simulink model "subCalc"  (R2016b)
settings: Solver=VariableStepAuto  StartTime=0.0  StopTime=10.0  RelTol=1e-3
settings Model: Creator=Radwa  LastModifiedBy=Radwa

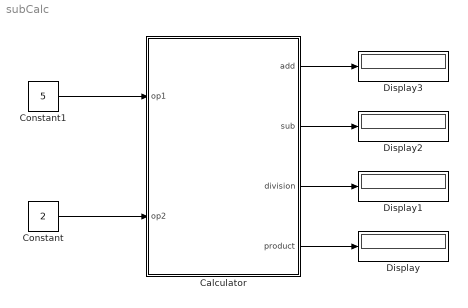
== system subCalc ==
  Calculator : Subsystem
  Constant : Constant  Value=2
  Constant1 : Constant  Value=5
  Display{,1..3} (4 alike) : Display
  wires:
  Constant1/1 -> Calculator/1(op1)
  Constant/1 -> Calculator/2(op2)
  Calculator/1(add) -> Display3/1
  Calculator/2(sub) -> Display2/1
  Calculator/3(division) -> Display1/1
  Calculator/4(product) -> Display/1

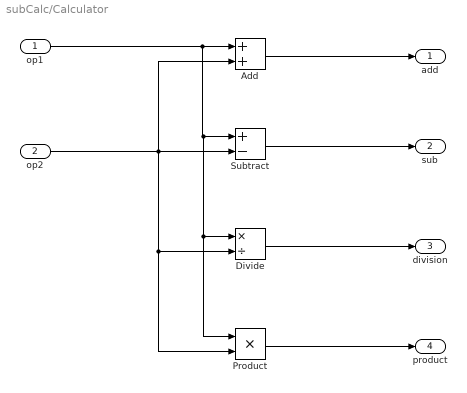
== system subCalc/Calculator ==
  op1 : Inport
  op2 : Inport  Port=2
  Add : Sum
  Divide : Product  Inputs=*/
  Product : Product
  Subtract : Sum  Inputs=+-
  add : Outport
  sub : Outport  Port=2
  division : Outport  Port=3
  product : Outport  Port=4
  wires:
  Add/1 -> add/1
  Subtract/1 -> sub/1
  Divide/1 -> division/1
  op1/1 -> Product/1, Divide/1, Subtract/1, Add/1
  Product/1 -> product/1
  op2/1 -> Product/2, Divide/2, Add/2, Subtract/2
